simulink model "test7_blocks_named_port_diff"  (R2016b)
settings: Solver=VariableStepAuto  StartTime=0.0  StopTime=10.0  RelTol=1e-3
settings Model: Creator=gm  LastModifiedBy=gm

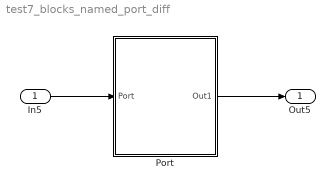
== system test7_blocks_named_port_diff ==
  In5 : Inport
  Port : Subsystem
  Out5 : Outport
  wires:
  In5/1 -> Port/1(Port)
  Port/1(Out1) -> Out5/1

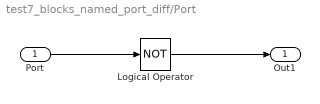
== system test7_blocks_named_port_diff/Port ==
  Port : Inport
  Logical Operator : Logic  Operator=NOT  AllPortsSameDT=off  OutDataTypeStr=boolean
  Out1 : Outport
  wires:
  Port/1 -> Logical Operator/1
  Logical Operator/1 -> Out1/1
